simulink model "matlab_arduino"  (R2016a)
settings: Solver=ode45  StartTime=0.0  StopTime=5  FixedStep=0.001  RelTol=1e-3
libraries: arduino_io_lib x6
settings Model: Creator=Gabriel  LastModifiedBy=Felippe
settings DataIOCC: LimitDataPoints=on  SaveFormat=Array
settings DebuggingCC: UnderspecifiedInitializationDetection=Classic  MergeDetectMultiDrivingBlocksExec=none  SolverPrmCheckMsg=warning  StateNameClashWarn=warning
settings HardwareCC: ProdBitPerPointer=32  ProdLargestAtomicFloat=None  ProdIntDivRoundTo=Undefined  ProdEndianess=Unspecified  ProdWordSize=32  ProdHWDeviceType=32-bit Generic
settings ModelReferenceCC: PropagateSignalLabelsOutOfModel=off
settings ConfigComp: CovModelRefEnable=Off

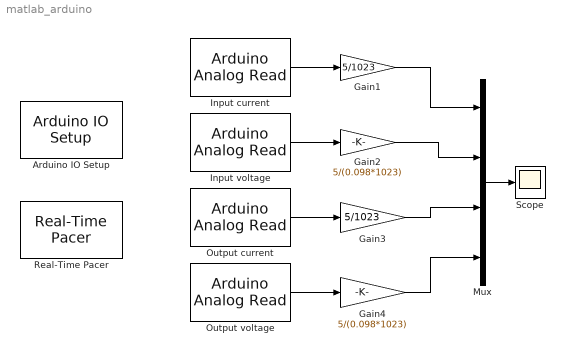
== system matlab_arduino ==
  Arduino IO Setup : arduino_io_lib/Arduino IO Setup  Priority=3  arduinoVar=Temporary arduino variable: Arduino1  workspaceVarName=a  comPort=COM5
  Gain1 : Gain  Gain=5/1023
  Gain2 : Gain  Gain=5/(0.098*1023)
  Gain3 : Gain  Gain=5/1023
  Gain4 : Gain  Gain=5/(0.098*1023)
  Input current : arduino_io_lib/Arduino Analog Read  arduinoVar=Temporary arduino variable: Arduino1  arduinoPin=4  T=0.02
  Input voltage : arduino_io_lib/Arduino Analog Read  arduinoVar=Temporary arduino variable: Arduino1  arduinoPin=5  T=0.02
  Mux : Mux
  Output current : arduino_io_lib/Arduino Analog Read  arduinoVar=Temporary arduino variable: Arduino1  arduinoPin=2  T=0.02
  Output voltage : arduino_io_lib/Arduino Analog Read  arduinoVar=Temporary arduino variable: Arduino1  arduinoPin=3  T=0.02
  Real-Time Pacer : arduino_io_lib/Real-Time Pacer  simTimePerRealTime=1
  Scope : Scope
  wires:
  Mux/1 -> Scope/1
  Input current/1 -> Gain1/1
  Gain1/1 -> Mux/1
  Output current/1 -> Gain3/1
  Output voltage/1 -> Gain4/1
  Gain3/1 -> Mux/3
  Gain4/1 -> Mux/4
  Input voltage/1 -> Gain2/1
  Gain2/1 -> Mux/2
